simulink model "EOM_oceancurrents"  (R2023b)
settings: Solver=ode45  StartTime=0.0  StopTime=100  RelTol=1e-3
values from neighbouring files (symbols this model uses):
  beta_w = 0    [EOM_input.m]
  CM = 2.909*10^-5    (= 2.909e-05)    [dcdata.m]
  flow = [a_c;b_c;speed_c]    [EOM_input.m]
  Jm = 6.24*10^-4    (= 0.000624)    [dcdata.m]
  Kb = 1.7629*10^-2    (= 0.017629)    [dcdata.m]
  Kt = 1.7629*10^-2    (= 0.017629)    [dcdata.m]
  La = 0.28    [dcdata.m]
  M = M_a + M_rb    [EOM_input.m]    (also in Mechatronics (1).m; Mechatronics.m)
  Ra = 0.22680    (= 0.2268)    [dcdata.m]
  tau_r = -T1*cos(alpha1)*0.065+T2*cos(alpha1)*0.35+T2*cos(alpha2)-T2*sin(alpha2)+Tb*0.35    [EOM_input.m]    (also in Mechatronics (1).m; Mechatronics.m)
  tau_u = T1*cos(alpha1)+T2*cos(alpha2)    [EOM_input.m]    (also in Mechatronics (1).m; Mechatronics.m)
  tau_v = T1*sin(alpha1)+T2*sin(alpha2)+Tb    [EOM_input.m]    (also in Mechatronics (1).m = T1*sin(alpha1)+T2*sin(alpha2); Mechatronics.m)
  Trat = Ia*Kt    (= 0.158661)    [dcdata.m]
  vw = 0    [EOM_input.m]
  wm = 564.9    [dcdata.m]
undefined symbols (not defined in the file or in its folder): current_magnitude_percentage, eta_req_global, eta_start_local, T_all
libraries: slpidlib x5
settings Model: Creator=helle  LastModifiedBy=chris

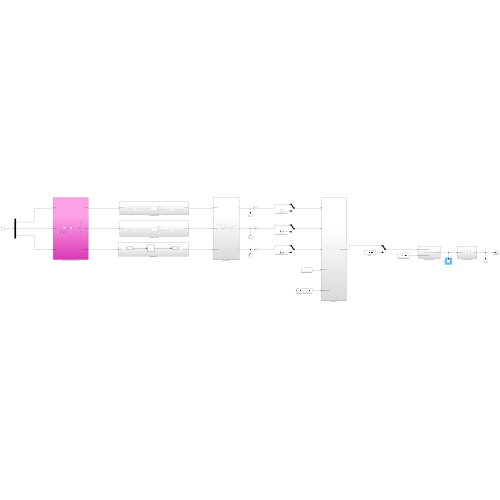
[thumbnail: Simulink's stored preview of the top-level diagram]
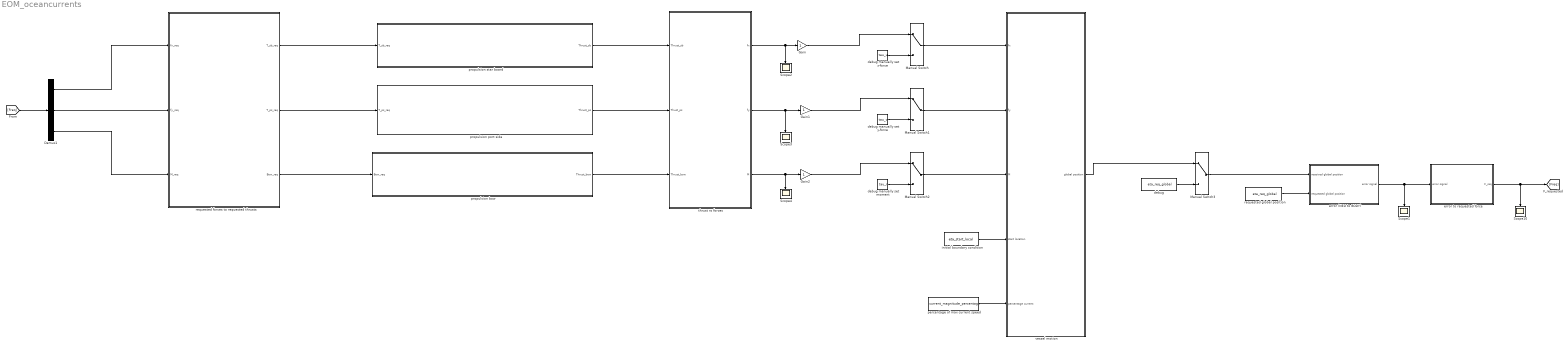
== system EOM_oceancurrents ==
  Demux1 : Demux  Outputs=3
  Gain : Gain
  Gain1 : Gain
  Gain2 : Gain
  Manual Switch{,1..3} (4 alike) : ManualSwitch
  Scope{1..4,10} (5 alike) : Scope
  debug : Constant  Value=eta_req_global
  debug manually set moment : Constant  Value=tau_r
  debug manually set x-force : Constant  Value=tau_u
  debug manually set y-force : Constant  Value=tau_v
  error (NED to BODY) : Subsystem
  error to requested force : Subsystem
  initial boundary condition : Constant  Value=eta_start_local
  percentage of max current speed : Constant  Value=current_magnitude_percentage
  propulsion bow : Subsystem
  propulsion port side : Subsystem
  propulsion star board : Subsystem
  requested forces to requested thrusts : Subsystem
  requested global position : Constant  Value=eta_req_global
  thrust ro forces : Subsystem
  vessel motion : Subsystem
  wires:
  Demux1/1 -> requested forces to requested thrusts/1(fx_req)
  Demux1/2 -> requested forces to requested thrusts/2(fy_req)
  Demux1/3 -> requested forces to requested thrusts/3(M_req)
  error to requested force/1(F_req) -> Scope10/1, [Freq]
  error (NED to BODY)/1(error signal) -> Scope1/1, error to requested force/1(error signal)
  thrust ro forces/1(fx) -> Scope2/1, Gain/1
  thrust ro forces/2(fy) -> Scope3/1, Gain1/1
  thrust ro forces/3(M) -> Scope4/1, Gain2/1
  propulsion bow/1(Thrust_bow) -> thrust ro forces/3(Thrust_bow)
  propulsion port side/1(Thrust_ps) -> thrust ro forces/2(Thust_ps)
  propulsion star board/1(Thrust_sb) -> thrust ro forces/1(Thrust_sb)
  requested forces to requested thrusts/1(T_sb_req) -> propulsion star board/1(T_sb_req)
  requested forces to requested thrusts/2(T_ps_req) -> propulsion port side/1(T_ps_req)
  requested forces to requested thrusts/3(Bow_req) -> propulsion bow/1(Bow_req)
  requested global position/1 -> error (NED to BODY)/2(requested global position)
  initial boundary condition/1 -> vessel motion/4(start location)
  [Freq] -> Demux1/1
  percentage of max current speed/1 -> vessel motion/5(percentage current)
  Manual Switch/1 -> vessel motion/1(fx)
  Gain/1 -> Manual Switch/1
  Manual Switch1/1 -> vessel motion/2(fy)
  Manual Switch2/1 -> vessel motion/3(M)
  Gain1/1 -> Manual Switch1/1
  Gain2/1 -> Manual Switch2/1
  debug manually set x-force/1 -> Manual Switch/2
  debug manually set y-force/1 -> Manual Switch1/2
  debug manually set moment/1 -> Manual Switch2/2
  Manual Switch3/1 -> error (NED to BODY)/1("received global position ")
  vessel motion/1(global position) -> Manual Switch3/1
  debug/1 -> Manual Switch3/2

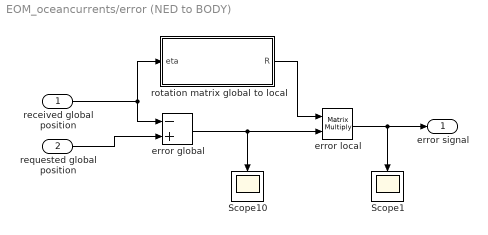
== system EOM_oceancurrents/error (NED to BODY) ==
  "received global position " : Inport
  requested global position : Inport  Port=2
  Scope1 : Scope
  Scope10 : Scope
  error global : Sum  Inputs=-+
  error local : Product  Multiplication=Matrix(*)
  rotation matrix global to local : MATLAB Function  TreatAsAtomicUnit=on
  error signal : Outport
  wires:
  "received global position "/1 -> rotation matrix global to local/1(eta), error global/1
  rotation matrix global to local/1(R) -> error local/1
  error local/1 -> Scope1/1, error signal/1
  requested global position/1 -> error global/2
  error global/1 -> Scope10/1, error local/2

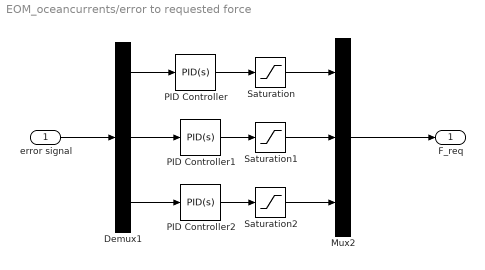
== system EOM_oceancurrents/error to requested force ==
  error signal : Inport
  Demux1 : Demux  Outputs=3
  Mux2 : Mux  Inputs=3
  PID Controller : slpidlib/PID Controller  Controller=PID  Form=Parallel  TimeDomain=Continuous-time  UseExternalTs=off  SampleTime=-1  IntegratorMethod=Forward Euler  FilterMethod=Forward Euler  ControllerParametersSource=internal  P=174.233635027511  I=4.06069558202177  UseKiTs=off  D=340.187698975111  N=319.667439985533  UseFilter=on  TunerSelectOption=Transfer Function Based (PID Tuner App)  InitialConditionSource=internal  InitialConditionForIntegrator=0  InitialConditionForFilter=0  DifferentiatorICPrevScaledInput=0  ExternalReset=none  TrackingMode=off  Kt=1  LimitOutput=off  SatLimitsSource=internal  UpperSaturationLimit=inf  LowerSaturationLimit=-inf  LinearizeAsGain=on  AntiWindupMode=none  Kb=1  LimitIntegrator=off  UpperIntegratorSaturationLimit=inf  LowerIntegratorSaturationLimit=-inf  POutMin=[]  POutMax=[]  IOutMin=[]  IOutMax=[]  DOutMin=[]  DOutMax=[]  NOutMin=[]  NOutMax=[]  SumOutMin=[]  SumOutMax=[]  SaturationOutMin=[]  SaturationOutMax=[]  PParamMin=[]  PParamMax=[]  IParamMin=[]  IParamMax=[]  DParamMin=[]  DParamMax=[]  NParamMin=[]  NParamMax=[]  KbParamMin=[]  KbParamMax=[]  KtParamMin=[]  KtParamMax=[]  KbOutMin=[]  KbOutMax=[]  KtOutMin=[]  KtOutMax=[]  IntegratorOutMin=[]  IntegratorOutMax=[]  FilterOutMin=[]  FilterOutMax=[]  SumI1OutMin=[]  SumI1OutMax=[]  SumI2OutMin=[]  SumI2OutMax=[]  SumI3OutMin=[]  SumI3OutMax=[]  SumI4OutMin=[]  SumI4OutMax=[]  SumDOutMin=[]  SumDOutMax=[]  DifferentiatorOutMin=[]  DifferentiatorOutMax=[]  FilterDiffOutCoefMin=[]  FilterDiffOutCoefMax=[]  ReciprocalOutMin=[]  ReciprocalOutMax=[]  SumDenOutMin=[]  SumDenOutMax=[]  SumNumOutMin=[]  SumNumOutMax=[]  DivideOutMin=[]  DivideOutMax=[]  UdiffTsProdOutMin=[]  UdiffTsProdOutMax=[]  NTsProdOutMin=[]  NTsProdOutMax=[]  UintegralTsProdOutMin=[]  UintegralTsProdOutMax=[]  UngainTsProdOutMin=[]  UngainTsProdOutMax=[]  ClampingZeroOutDataTypeStr=Inherit: Inherit via back propagation  ClampingZeroOutMin=[]  ClampingZeroOutMax=[]  FilterDenConstantOutDataTypeStr=Inherit: Inherit via back propagation  FilterDenConstantOutMin=[]  FilterDenConstantOutMax=[]  PCopyOutDataTypeStr=Inherit: Inherit via back propagation  PCopyOutMin=[]  PCopyOutMax=[]  NCopyOutDataTypeStr=Inherit: Inherit via back propagation  NCopyOutMin=[]  NCopyOutMax=[]  IntegratorContinuousStateAttributes=''  IntegratorStateMustResolveToSignalObject=off  IntegratorRTWStateStorageClass=Auto  FilterContinuousStateAttributes=''  FilterStateMustResolveToSignalObject=off  FilterRTWStateStorageClass=Auto  ParallelPVariant=InternalParameters  IdealPVariant=Disabled  IVariant=InternalParameters  DVariant=InternalParameters  IntegratorVariant=Continuous  SatVariant=Disabled  AWVariant=Passthrough  PCopyVariant=Disabled  TRVariant=Disabled  FdbkBlocksVariant=Forward  IdealPFdbkVariant=Disabled  SatFdbkVariant=Disabled  DerivativeFilterVariant=ContFilter  NVariant=InternalParameters  NCopyVariant=Disabled  FilterICVariant=InternalICsFilter  IntegratorICVariant=InternalICs  ExternalResetVariant=Disabled  TRSumVariant=Passthrough  SumFdbkVariant=Disabled  SumVariant=Sum_PID  TsampFilterVariant=InternalTs  TsampNgainVariant=Passthrough  TsampIntegralVariant=Disabled_SignalSpec  ExternalSaturationOutDataTypeStr=Inherit: Same as second input
  PID Controller1 : slpidlib/PID Controller  Controller=PID  Form=Parallel  TimeDomain=Continuous-time  UseExternalTs=off  SampleTime=-1  IntegratorMethod=Forward Euler  FilterMethod=Forward Euler  ControllerParametersSource=internal  P=97592.719586186  I=747986.305690658  UseKiTs=off  D=3078.78047810734  N=541.472412487083  UseFilter=on  TunerSelectOption=Transfer Function Based (PID Tuner App)  InitialConditionSource=internal  InitialConditionForIntegrator=0  InitialConditionForFilter=0  DifferentiatorICPrevScaledInput=0  ExternalReset=none  TrackingMode=off  Kt=1  LimitOutput=off  SatLimitsSource=internal  UpperSaturationLimit=inf  LowerSaturationLimit=-inf  LinearizeAsGain=on  AntiWindupMode=none  Kb=1  LimitIntegrator=off  UpperIntegratorSaturationLimit=inf  LowerIntegratorSaturationLimit=-inf  POutMin=[]  POutMax=[]  IOutMin=[]  IOutMax=[]  DOutMin=[]  DOutMax=[]  NOutMin=[]  NOutMax=[]  SumOutMin=[]  SumOutMax=[]  SaturationOutMin=[]  SaturationOutMax=[]  PParamMin=[]  PParamMax=[]  IParamMin=[]  IParamMax=[]  DParamMin=[]  DParamMax=[]  NParamMin=[]  NParamMax=[]  KbParamMin=[]  KbParamMax=[]  KtParamMin=[]  KtParamMax=[]  KbOutMin=[]  KbOutMax=[]  KtOutMin=[]  KtOutMax=[]  IntegratorOutMin=[]  IntegratorOutMax=[]  FilterOutMin=[]  FilterOutMax=[]  SumI1OutMin=[]  SumI1OutMax=[]  SumI2OutMin=[]  SumI2OutMax=[]  SumI3OutMin=[]  SumI3OutMax=[]  SumI4OutMin=[]  SumI4OutMax=[]  SumDOutMin=[]  SumDOutMax=[]  DifferentiatorOutMin=[]  DifferentiatorOutMax=[]  FilterDiffOutCoefMin=[]  FilterDiffOutCoefMax=[]  ReciprocalOutMin=[]  ReciprocalOutMax=[]  SumDenOutMin=[]  SumDenOutMax=[]  SumNumOutMin=[]  SumNumOutMax=[]  DivideOutMin=[]  DivideOutMax=[]  UdiffTsProdOutMin=[]  UdiffTsProdOutMax=[]  NTsProdOutMin=[]  NTsProdOutMax=[]  UintegralTsProdOutMin=[]  UintegralTsProdOutMax=[]  UngainTsProdOutMin=[]  UngainTsProdOutMax=[]  ClampingZeroOutDataTypeStr=Inherit: Inherit via back propagation  ClampingZeroOutMin=[]  ClampingZeroOutMax=[]  FilterDenConstantOutDataTypeStr=Inherit: Inherit via back propagation  FilterDenConstantOutMin=[]  FilterDenConstantOutMax=[]  PCopyOutDataTypeStr=Inherit: Inherit via back propagation  PCopyOutMin=[]  PCopyOutMax=[]  NCopyOutDataTypeStr=Inherit: Inherit via back propagation  NCopyOutMin=[]  NCopyOutMax=[]  IntegratorContinuousStateAttributes=''  IntegratorStateMustResolveToSignalObject=off  IntegratorRTWStateStorageClass=Auto  FilterContinuousStateAttributes=''  FilterStateMustResolveToSignalObject=off  FilterRTWStateStorageClass=Auto  ParallelPVariant=InternalParameters  IdealPVariant=Disabled  IVariant=InternalParameters  DVariant=InternalParameters  IntegratorVariant=Continuous  SatVariant=Disabled  AWVariant=Passthrough  PCopyVariant=Disabled  TRVariant=Disabled  FdbkBlocksVariant=Forward  IdealPFdbkVariant=Disabled  SatFdbkVariant=Disabled  DerivativeFilterVariant=ContFilter  NVariant=InternalParameters  NCopyVariant=Disabled  FilterICVariant=InternalICsFilter  IntegratorICVariant=InternalICs  ExternalResetVariant=Disabled  TRSumVariant=Passthrough  SumFdbkVariant=Disabled  SumVariant=Sum_PID  TsampFilterVariant=InternalTs  TsampNgainVariant=Passthrough  TsampIntegralVariant=Disabled_SignalSpec  ExternalSaturationOutDataTypeStr=Inherit: Same as second input
  PID Controller2 : slpidlib/PID Controller  Controller=PID  Form=Parallel  TimeDomain=Continuous-time  UseExternalTs=off  SampleTime=-1  IntegratorMethod=Forward Euler  FilterMethod=Forward Euler  ControllerParametersSource=internal  P=10.3561114578664  I=0.45191825910223  UseKiTs=off  D=53.5979577299415  N=151.545098117795  UseFilter=on  TunerSelectOption=Transfer Function Based (PID Tuner App)  InitialConditionSource=internal  InitialConditionForIntegrator=0  InitialConditionForFilter=0  DifferentiatorICPrevScaledInput=0  ExternalReset=none  TrackingMode=off  Kt=1  LimitOutput=off  SatLimitsSource=internal  UpperSaturationLimit=inf  LowerSaturationLimit=-inf  LinearizeAsGain=on  AntiWindupMode=none  Kb=1  LimitIntegrator=off  UpperIntegratorSaturationLimit=inf  LowerIntegratorSaturationLimit=-inf  POutMin=[]  POutMax=[]  IOutMin=[]  IOutMax=[]  DOutMin=[]  DOutMax=[]  NOutMin=[]  NOutMax=[]  SumOutMin=[]  SumOutMax=[]  SaturationOutMin=[]  SaturationOutMax=[]  PParamMin=[]  PParamMax=[]  IParamMin=[]  IParamMax=[]  DParamMin=[]  DParamMax=[]  NParamMin=[]  NParamMax=[]  KbParamMin=[]  KbParamMax=[]  KtParamMin=[]  KtParamMax=[]  KbOutMin=[]  KbOutMax=[]  KtOutMin=[]  KtOutMax=[]  IntegratorOutMin=[]  IntegratorOutMax=[]  FilterOutMin=[]  FilterOutMax=[]  SumI1OutMin=[]  SumI1OutMax=[]  SumI2OutMin=[]  SumI2OutMax=[]  SumI3OutMin=[]  SumI3OutMax=[]  SumI4OutMin=[]  SumI4OutMax=[]  SumDOutMin=[]  SumDOutMax=[]  DifferentiatorOutMin=[]  DifferentiatorOutMax=[]  FilterDiffOutCoefMin=[]  FilterDiffOutCoefMax=[]  ReciprocalOutMin=[]  ReciprocalOutMax=[]  SumDenOutMin=[]  SumDenOutMax=[]  SumNumOutMin=[]  SumNumOutMax=[]  DivideOutMin=[]  DivideOutMax=[]  UdiffTsProdOutMin=[]  UdiffTsProdOutMax=[]  NTsProdOutMin=[]  NTsProdOutMax=[]  UintegralTsProdOutMin=[]  UintegralTsProdOutMax=[]  UngainTsProdOutMin=[]  UngainTsProdOutMax=[]  ClampingZeroOutDataTypeStr=Inherit: Inherit via back propagation  ClampingZeroOutMin=[]  ClampingZeroOutMax=[]  FilterDenConstantOutDataTypeStr=Inherit: Inherit via back propagation  FilterDenConstantOutMin=[]  FilterDenConstantOutMax=[]  PCopyOutDataTypeStr=Inherit: Inherit via back propagation  PCopyOutMin=[]  PCopyOutMax=[]  NCopyOutDataTypeStr=Inherit: Inherit via back propagation  NCopyOutMin=[]  NCopyOutMax=[]  IntegratorContinuousStateAttributes=''  IntegratorStateMustResolveToSignalObject=off  IntegratorRTWStateStorageClass=Auto  FilterContinuousStateAttributes=''  FilterStateMustResolveToSignalObject=off  FilterRTWStateStorageClass=Auto  ParallelPVariant=InternalParameters  IdealPVariant=Disabled  IVariant=InternalParameters  DVariant=InternalParameters  IntegratorVariant=Continuous  SatVariant=Disabled  AWVariant=Passthrough  PCopyVariant=Disabled  TRVariant=Disabled  FdbkBlocksVariant=Forward  IdealPFdbkVariant=Disabled  SatFdbkVariant=Disabled  DerivativeFilterVariant=ContFilter  NVariant=InternalParameters  NCopyVariant=Disabled  FilterICVariant=InternalICsFilter  IntegratorICVariant=InternalICs  ExternalResetVariant=Disabled  TRSumVariant=Passthrough  SumFdbkVariant=Disabled  SumVariant=Sum_PID  TsampFilterVariant=InternalTs  TsampNgainVariant=Passthrough  TsampIntegralVariant=Disabled_SignalSpec  ExternalSaturationOutDataTypeStr=Inherit: Same as second input
  Saturation : Saturate  UpperLimit=2.5  LowerLimit=-2.5
  Saturation1 : Saturate  UpperLimit=2.5  LowerLimit=-2.5
  Saturation2 : Saturate  UpperLimit=2.5  LowerLimit=-2.5
  F_req : Outport
  wires:
  error signal/1 -> Demux1/1
  Demux1/1 -> PID Controller/1
  PID Controller1/1 -> Saturation1/1
  Saturation/1 -> Mux2/1
  Saturation2/1 -> Mux2/3
  Mux2/1 -> F_req/1
  PID Controller/1 -> Saturation/1
  Demux1/2 -> PID Controller1/1
  Saturation1/1 -> Mux2/2
  Demux1/3 -> PID Controller2/1
  PID Controller2/1 -> Saturation2/1

== system EOM_oceancurrents/propulsion bow ==
  Bow_req : Inport
  Saturation : Saturate  UpperLimit=2  LowerLimit=-2
  Thrust_bow : Outport
  wires:
  Saturation/1 -> Thrust_bow/1
  Bow_req/1 -> Saturation/1

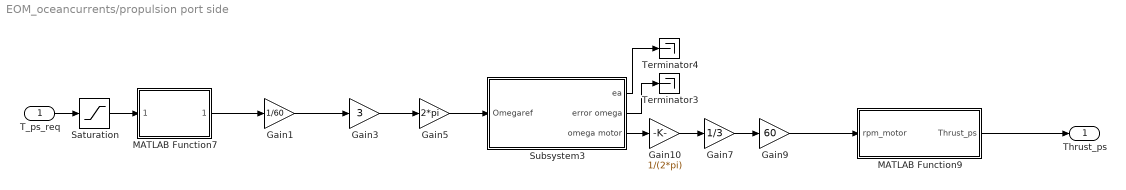
== system EOM_oceancurrents/propulsion port side ==
  T_ps_req : Inport
  Gain1 : Gain  Gain=1/60
  Gain10 : Gain  Gain=1/(2*pi)
  Gain3 : Gain  Gain=3
  Gain5 : Gain  Gain=2*pi
  Gain7 : Gain  Gain=1/3
  Gain9 : Gain  Gain=60
  MATLAB Function7 : MATLAB Function  TreatAsAtomicUnit=on
  MATLAB Function9 : MATLAB Function  TreatAsAtomicUnit=on
  Saturation : Saturate  UpperLimit=3  LowerLimit=-3
  Subsystem3 : Subsystem
  Terminator3 : Terminator
  Terminator4 : Terminator
  Thrust_ps : Outport
  wires:
  Gain9/1 -> MATLAB Function9/1(rpm_motor)
  T_ps_req/1 -> Saturation/1
  Gain5/1 -> Subsystem3/1(Omegaref)
  Gain10/1 -> Gain7/1
  Gain7/1 -> Gain9/1
  Gain3/1 -> Gain5/1
  MATLAB Function7/1(rpmreq) -> Gain1/1
  Subsystem3/3(omega motor) -> Gain10/1
  MATLAB Function9/1(Thrust_ps) -> Thrust_ps/1
  Gain1/1 -> Gain3/1
  Subsystem3/2(error omega) -> Terminator3/1
  Subsystem3/1(ea) -> Terminator4/1
  Saturation/1 -> MATLAB Function7/1(T_ps_req)

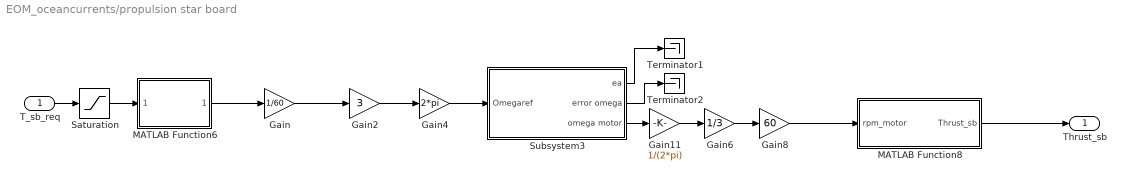
== system EOM_oceancurrents/propulsion star board ==
  T_sb_req : Inport
  Gain : Gain  Gain=1/60
  Gain11 : Gain  Gain=1/(2*pi)
  Gain2 : Gain  Gain=3
  Gain4 : Gain  Gain=2*pi
  Gain6 : Gain  Gain=1/3
  Gain8 : Gain  Gain=60
  MATLAB Function6 : MATLAB Function  TreatAsAtomicUnit=on
  MATLAB Function8 : MATLAB Function  TreatAsAtomicUnit=on
  Saturation : Saturate  UpperLimit=3  LowerLimit=-3
  Subsystem3 : Subsystem
  Terminator1 : Terminator
  Terminator2 : Terminator
  Thrust_sb : Outport
  wires:
  MATLAB Function6/1(rpmreq) -> Gain/1
  T_sb_req/1 -> Saturation/1
  Subsystem3/3(omega motor) -> Gain11/1
  Gain6/1 -> Gain8/1
  Subsystem3/1(ea) -> Terminator1/1
  Gain2/1 -> Gain4/1
  Gain11/1 -> Gain6/1
  Gain4/1 -> Subsystem3/1(Omegaref)
  Gain/1 -> Gain2/1
  MATLAB Function8/1(Thrust_sb) -> Thrust_sb/1
  Gain8/1 -> MATLAB Function8/1(rpm_motor)
  Subsystem3/2(error omega) -> Terminator2/1
  Saturation/1 -> MATLAB Function6/1(T_sb_req)

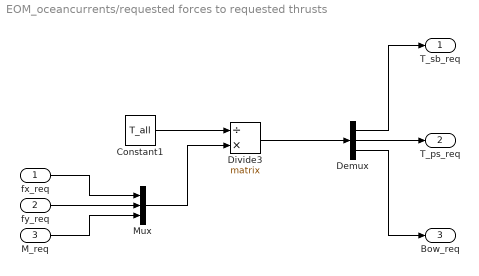
== system EOM_oceancurrents/requested forces to requested thrusts ==
  fx_req : Inport
  fy_req : Inport  Port=2
  M_req : Inport  Port=3
  Constant1 : Constant  Value=T_all
  Demux : Demux  Outputs=3
  Divide3 : Product  Inputs=/*  Multiplication=Matrix(*)
  Mux : Mux  Inputs=3
  T_sb_req : Outport
  T_ps_req : Outport  Port=2
  Bow_req : Outport  Port=3
  wires:
  Demux/1 -> T_sb_req/1
  Mux/1 -> Divide3/2
  Demux/3 -> Bow_req/1
  M_req/1 -> Mux/3
  fy_req/1 -> Mux/2
  Divide3/1 -> Demux/1
  Demux/2 -> T_ps_req/1
  Constant1/1 -> Divide3/1
  fx_req/1 -> Mux/1

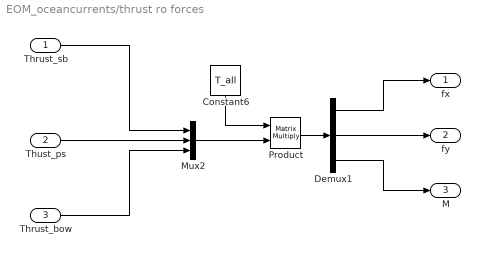
== system EOM_oceancurrents/thrust ro forces ==
  Thrust_sb : Inport
  Thust_ps : Inport  Port=2
  Thrust_bow : Inport  Port=3
  Constant6 : Constant  Value=T_all
  Demux1 : Demux  Outputs=3
  Mux2 : Mux  Inputs=3
  Product : Product  Multiplication=Matrix(*)
  fx : Outport
  fy : Outport  Port=2
  M : Outport  Port=3
  wires:
  Thrust_bow/1 -> Mux2/3
  Thrust_sb/1 -> Mux2/1
  Demux1/1 -> fx/1
  Mux2/1 -> Product/2
  Thust_ps/1 -> Mux2/2
  Demux1/3 -> M/1
  Demux1/2 -> fy/1
  Constant6/1 -> Product/1
  Product/1 -> Demux1/1

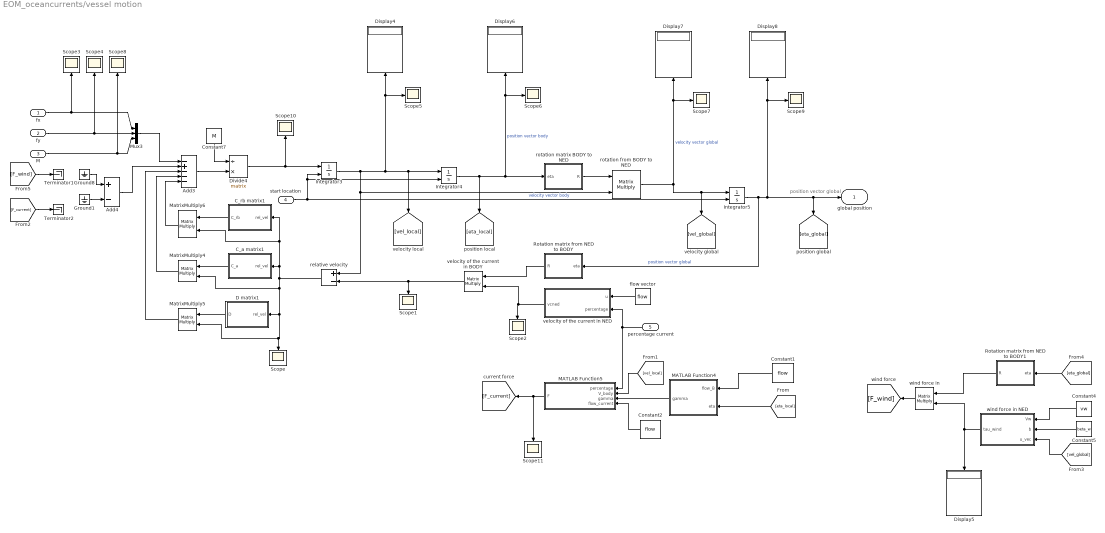
== system EOM_oceancurrents/vessel motion ==
  note: position vector global
  fx : Inport
  fy : Inport  Port=2
  M : Inport  Port=3
  start location : Inport  Port=4
  percentage current : Inport  Port=5
  Add3 : Sum  Inputs=-+---
  Add4 : Sum  Inputs=+-
  C_a matrix1 : MATLAB Function  TreatAsAtomicUnit=on
  C_rb matrix1 : MATLAB Function  TreatAsAtomicUnit=on
  Constant1 : Constant  Value=flow
  Constant2 : Constant  Value=flow
  Constant4 : Constant  Value=vw
  Constant5 : Constant  Value=beta_w
  Constant7 : Constant  Value=M
  D matrix1 : MATLAB Function  TreatAsAtomicUnit=on
  Display{4..8} (5 alike) : Display
  Divide4 : Product  Inputs=/*  Multiplication=Matrix(*)
  Ground1 : Ground
  Ground8 : Ground
  Integrator3 : Integrator  InitialConditionSource=external
  Integrator4 : Integrator  InitialConditionSource=external
  Integrator5 : Integrator  InitialConditionSource=external
  MATLAB Function4 : MATLAB Function  TreatAsAtomicUnit=on
  MATLAB Function5 : MATLAB Function  TreatAsAtomicUnit=on
  MatrixMultiply4 : Product  Multiplication=Matrix(*)
  MatrixMultiply5 : Product  Multiplication=Matrix(*)
  MatrixMultiply6 : Product  Multiplication=Matrix(*)
  Mux3 : Mux  Inputs=3
  Rotation matrix from NED to BODY : MATLAB Function  TreatAsAtomicUnit=on
  Rotation matrix from NED to BODY1 : MATLAB Function  TreatAsAtomicUnit=on
  Scope{,1..11} (12 alike) : Scope
  Terminator1 : Terminator
  Terminator2 : Terminator
  flow vector : Constant  Value=flow
  relative velocity : Sum  Inputs=+-
  rotation from BODY to NED : Product  Multiplication=Matrix(*)
  rotation matrix BODY to NED : MATLAB Function  TreatAsAtomicUnit=on
  velocity of the current in BODY : Product  Inputs=**  Multiplication=Matrix(*)
  velocity of the current in NED : MATLAB Function  TreatAsAtomicUnit=on
  "wind force in " : Product  Inputs=**  Multiplication=Matrix(*)
  wind force in NED : MATLAB Function  TreatAsAtomicUnit=on
  global position : Outport
  wires:
  Integrator3/1 -> Scope5/1, Display4/1, [vel_local], Integrator4/1, relative velocity/1, rotation from BODY to NED/2  "velocity vector body"
  rotation from BODY to NED/1 -> Scope7/1, Display7/1, [vel_global], Integrator5/1  "velocity vector global"
  Divide4/1 -> Scope10/1, Integrator3/1
  relative velocity/1 -> Scope/1, MatrixMultiply5/2, D matrix1/1(rel_vel), MatrixMultiply4/2, C_a matrix1/1(rel_vel), C_rb matrix1/1(rel_vel), MatrixMultiply6/2
  Integrator5/1 -> [eta_global], global position/1, Display8/1, Scope9/1, Rotation matrix from NED to BODY/1(eta)  "position vector global"
  Integrator4/1 -> Scope6/1, Display6/1, rotation matrix BODY to NED/1(eta), [eta_local]  "position vector body"
  C_rb matrix1/1(C_rb) -> MatrixMultiply6/1
  Ground8/1 -> Add4/1
  MatrixMultiply4/1 -> Add3/4
  MatrixMultiply6/1 -> Add3/5
  rotation matrix BODY to NED/1(R) -> rotation from BODY to NED/1
  D matrix1/1(D) -> MatrixMultiply5/1
  C_a matrix1/1(C_a) -> MatrixMultiply4/1
  Mux3/1 -> Add3/1
  MatrixMultiply5/1 -> Add3/3
  Rotation matrix from NED to BODY/1(R) -> velocity of the current in BODY/1
  Constant7/1 -> Divide4/1
  Add3/1 -> Divide4/2
  Add4/1 -> Add3/2
  flow vector/1 -> velocity of the current in NED/1(u)
  velocity of the current in BODY/1 -> Scope1/1, relative velocity/2
  fy/1 -> Scope4/1, Mux3/2
  fx/1 -> Scope3/1, Mux3/1
  M/1 -> Scope8/1, Mux3/3
  MATLAB Function4/1(gamma) -> MATLAB Function5/3(gamma)
  [eta_local] -> MATLAB Function4/2(eta)
  Constant1/1 -> MATLAB Function4/1(flow_B)
  Constant2/1 -> MATLAB Function5/4(flow_current)
  [vel_local] -> MATLAB Function5/2(V_body)
  MATLAB Function5/1(F) -> Scope11/1, [F_current]
  velocity of the current in NED/1(vcned) -> Scope2/1, velocity of the current in BODY/2
  Constant4/1 -> wind force in NED/1(Vw)
  "wind force in "/1 -> [F_wind]
  Constant5/1 -> wind force in NED/2(b)
  wind force in NED/1(tau_wind) -> Display5/1, "wind force in "/2
  [vel_global] -> wind force in NED/3(u_vec)
  [eta_global] -> Rotation matrix from NED to BODY1/1(eta)
  Rotation matrix from NED to BODY1/1(R) -> "wind force in "/1
  [F_wind] -> Terminator1/1
  start location/1 -> Integrator3/2, Integrator4/2, Integrator5/2
  percentage current/1 -> velocity of the current in NED/2(percentage), MATLAB Function5/1(percentage)
  [F_current] -> Terminator2/1
  Ground1/1 -> Add4/2

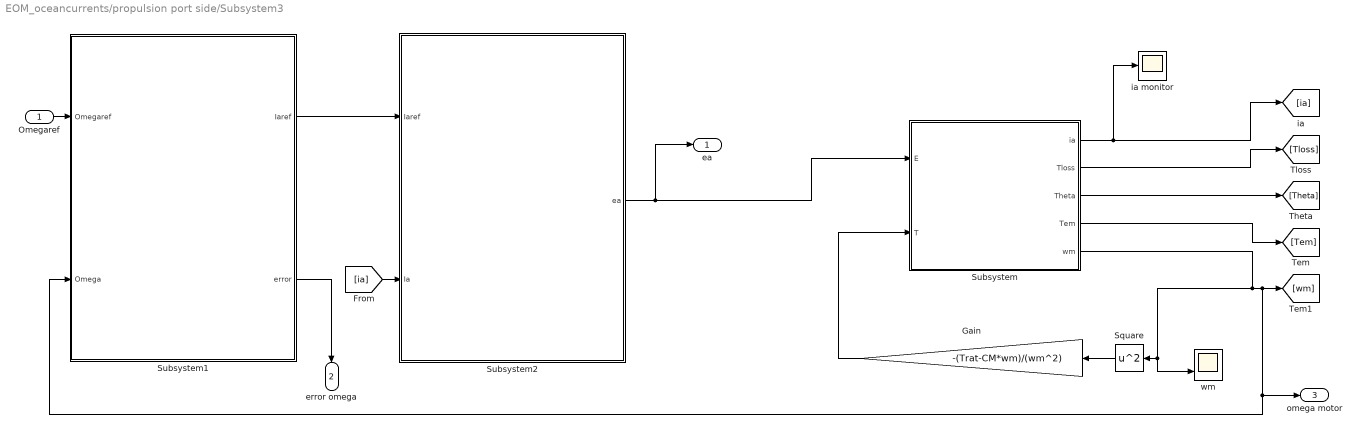
== system EOM_oceancurrents/propulsion port side/Subsystem3 ==
  Omegaref : Inport
  Gain : Gain  Gain=-(Trat-CM*wm)/(wm^2)
  Square : Math  Operator=square
  Subsystem : Subsystem
  Subsystem1 : Subsystem
  Subsystem2 : Subsystem
  ia monitor : Scope
  wm : Scope  NumInputPorts=2
  ea : Outport
  error omega : Outport  Port=2
  omega motor : Outport  Port=3
  wires:
  Subsystem/5(wm) -> omega motor/1, Subsystem1/2(Omega), [wm], Square/1, wm/2
  Gain/1 -> Subsystem/2(T)
  Subsystem/1(ia) -> ia monitor/1, [ia]
  Subsystem1/1(Iaref) -> Subsystem2/1(Iaref)
  Subsystem1/2(error) -> error omega/1
  Square/1 -> Gain/1
  Omegaref/1 -> Subsystem1/1(Omegaref)
  Subsystem2/1(ea) -> Subsystem/1(E), ea/1
  Subsystem/2(Tloss) -> [Tloss]
  Subsystem/3(Theta) -> [Theta]
  Subsystem/4(Tem) -> [Tem]
  [ia] -> Subsystem2/2(Ia)

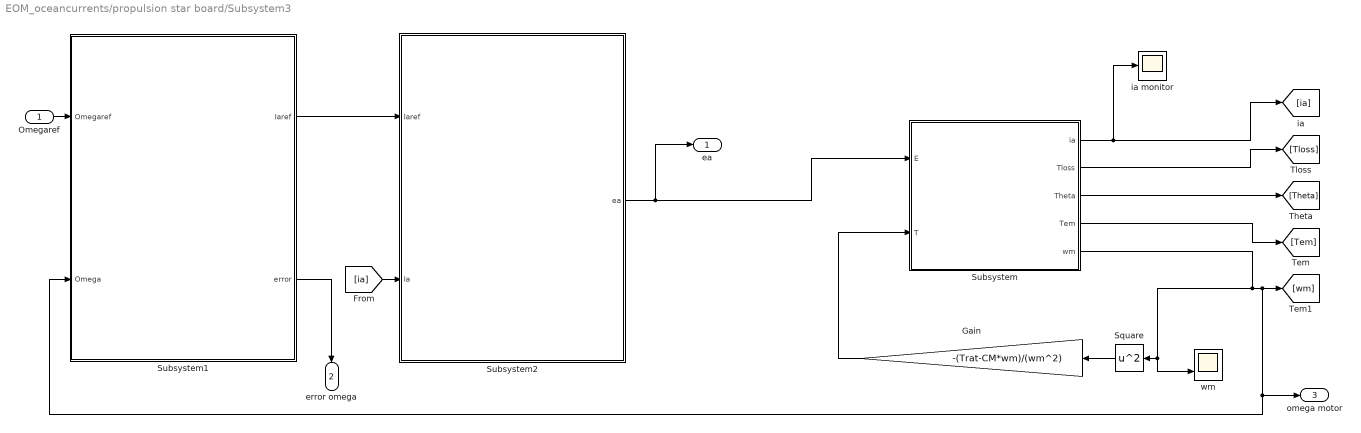
== system EOM_oceancurrents/propulsion star board/Subsystem3 ==
  Omegaref : Inport
  Gain : Gain  Gain=-(Trat-CM*wm)/(wm^2)
  Square : Math  Operator=square
  Subsystem : Subsystem
  Subsystem1 : Subsystem
  Subsystem2 : Subsystem
  ia monitor : Scope
  wm : Scope  NumInputPorts=2
  ea : Outport
  error omega : Outport  Port=2
  omega motor : Outport  Port=3
  wires:
  Subsystem/5(wm) -> omega motor/1, Subsystem1/2(Omega), [wm], Square/1, wm/2
  Gain/1 -> Subsystem/2(T)
  Subsystem/1(ia) -> ia monitor/1, [ia]
  Subsystem1/1(Iaref) -> Subsystem2/1(Iaref)
  Subsystem1/2(error) -> error omega/1
  Square/1 -> Gain/1
  Omegaref/1 -> Subsystem1/1(Omegaref)
  Subsystem2/1(ea) -> Subsystem/1(E), ea/1
  Subsystem/2(Tloss) -> [Tloss]
  Subsystem/3(Theta) -> [Theta]
  Subsystem/4(Tem) -> [Tem]
  [ia] -> Subsystem2/2(Ia)

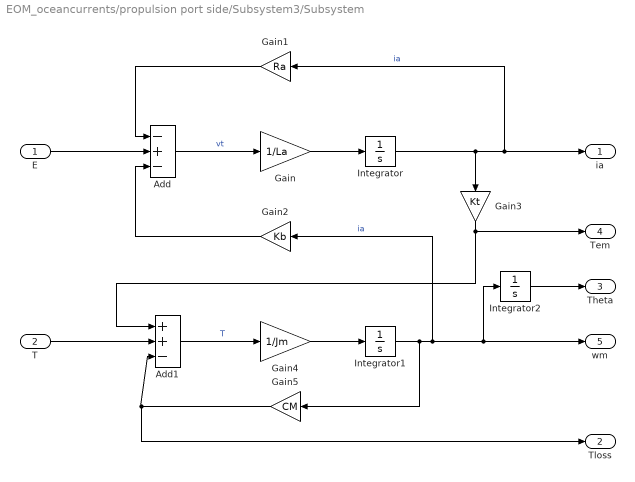
== system EOM_oceancurrents/propulsion port side/Subsystem3/Subsystem ==
  E : Inport
  T : Inport  Port=2
  Add : Sum  Inputs=-+-
  Add1 : Sum  Inputs=++-
  Gain : Gain  Gain=1/La
  Gain1 : Gain  Gain=Ra
  Gain2 : Gain  Gain=Kb
  Gain3 : Gain  Gain=Kt
  Gain4 : Gain  Gain=1/Jm
  Gain5 : Gain  Gain=CM
  Integrator : Integrator
  Integrator1 : Integrator
  Integrator2 : Integrator
  ia : Outport
  Tloss : Outport  Port=2
  Theta : Outport  Port=3
  Tem : Outport  Port=4
  wm : Outport  Port=5
  wires:
  Gain2/1 -> Add/3
  Gain/1 -> Integrator/1
  Integrator1/1 -> wm/1, Integrator2/1, Gain2/1, Gain5/1  "ia"
  Add1/1 -> Gain4/1  "T"
  Add/1 -> Gain/1  "vt"
  Gain1/1 -> Add/1
  Gain4/1 -> Integrator1/1
  Integrator/1 -> ia/1, Gain1/1, Gain3/1  "ia"
  Gain3/1 -> Add1/1, Tem/1
  Gain5/1 -> Tloss/1, Add1/3
  E/1 -> Add/2
  T/1 -> Add1/2
  Integrator2/1 -> Theta/1

== system EOM_oceancurrents/propulsion port side/Subsystem3/Subsystem1 ==
  Omegaref : Inport
  Omega : Inport  Port=2
  Add : Sum  Inputs=+-
  Gain : Gain  Gain=1/wm
  PID Controller : slpidlib/PID Controller  Controller=PID  Form=Ideal  TimeDomain=Continuous-time  UseExternalTs=off  SampleTime=-1  IntegratorMethod=Forward Euler  FilterMethod=Forward Euler  ControllerParametersSource=internal  P=99.1419908148733  I=0.405774649898487  UseKiTs=off  D=0.0328385363334431  N=5.23608118750105  UseFilter=on  TunerSelectOption=Transfer Function Based (PID Tuner App)  InitialConditionSource=internal  InitialConditionForIntegrator=0  InitialConditionForFilter=0  DifferentiatorICPrevScaledInput=0  ExternalReset=none  TrackingMode=off  Kt=1  LimitOutput=off  SatLimitsSource=internal  UpperSaturationLimit=inf  LowerSaturationLimit=-inf  LinearizeAsGain=on  AntiWindupMode=none  Kb=1  LimitIntegrator=off  UpperIntegratorSaturationLimit=inf  LowerIntegratorSaturationLimit=-inf  POutMin=[]  POutMax=[]  IOutMin=[]  IOutMax=[]  DOutMin=[]  DOutMax=[]  NOutMin=[]  NOutMax=[]  SumOutMin=[]  SumOutMax=[]  SaturationOutMin=[]  SaturationOutMax=[]  PParamMin=[]  PParamMax=[]  IParamMin=[]  IParamMax=[]  DParamMin=[]  DParamMax=[]  NParamMin=[]  NParamMax=[]  KbParamMin=[]  KbParamMax=[]  KtParamMin=[]  KtParamMax=[]  KbOutMin=[]  KbOutMax=[]  KtOutMin=[]  KtOutMax=[]  IntegratorOutMin=[]  IntegratorOutMax=[]  FilterOutMin=[]  FilterOutMax=[]  SumI1OutMin=[]  SumI1OutMax=[]  SumI2OutMin=[]  SumI2OutMax=[]  SumI3OutMin=[]  SumI3OutMax=[]  SumI4OutMin=[]  SumI4OutMax=[]  SumDOutMin=[]  SumDOutMax=[]  DifferentiatorOutMin=[]  DifferentiatorOutMax=[]  FilterDiffOutCoefMin=[]  FilterDiffOutCoefMax=[]  ReciprocalOutMin=[]  ReciprocalOutMax=[]  SumDenOutMin=[]  SumDenOutMax=[]  SumNumOutMin=[]  SumNumOutMax=[]  DivideOutMin=[]  DivideOutMax=[]  UdiffTsProdOutMin=[]  UdiffTsProdOutMax=[]  NTsProdOutMin=[]  NTsProdOutMax=[]  UintegralTsProdOutMin=[]  UintegralTsProdOutMax=[]  UngainTsProdOutMin=[]  UngainTsProdOutMax=[]  ClampingZeroOutDataTypeStr=Inherit: Inherit via back propagation  ClampingZeroOutMin=[]  ClampingZeroOutMax=[]  FilterDenConstantOutDataTypeStr=Inherit: Inherit via back propagation  FilterDenConstantOutMin=[]  FilterDenConstantOutMax=[]  PCopyOutDataTypeStr=Inherit: Inherit via back propagation  PCopyOutMin=[]  PCopyOutMax=[]  NCopyOutDataTypeStr=Inherit: Inherit via back propagation  NCopyOutMin=[]  NCopyOutMax=[]  IntegratorContinuousStateAttributes=''  IntegratorStateMustResolveToSignalObject=off  IntegratorRTWStateStorageClass=Auto  FilterContinuousStateAttributes=''  FilterStateMustResolveToSignalObject=off  FilterRTWStateStorageClass=Auto  ParallelPVariant=Passthrough  IdealPVariant=InternalParameters  IVariant=InternalParameters  DVariant=InternalParameters  IntegratorVariant=Continuous  SatVariant=Disabled  AWVariant=Passthrough  PCopyVariant=Disabled  TRVariant=Disabled  FdbkBlocksVariant=Forward  IdealPFdbkVariant=Disabled  SatFdbkVariant=Disabled  DerivativeFilterVariant=ContFilter  NVariant=InternalParameters  NCopyVariant=Disabled  FilterICVariant=InternalICsFilter  IntegratorICVariant=InternalICs  ExternalResetVariant=Disabled  TRSumVariant=Passthrough  SumFdbkVariant=Disabled  SumVariant=Sum_PID  TsampFilterVariant=InternalTs  TsampNgainVariant=Passthrough  TsampIntegralVariant=Disabled_SignalSpec  ExternalSaturationOutDataTypeStr=Inherit: Same as second input
  Saturation : Saturate
  Iaref : Outport
  error : Outport  Port=2
  wires:
  Omegaref/1 -> Add/1
  Omega/1 -> Add/2
  Add/1 -> Gain/1
  Gain/1 -> PID Controller/1, error/1
  Saturation/1 -> Iaref/1
  PID Controller/1 -> Saturation/1

== system EOM_oceancurrents/propulsion port side/Subsystem3/Subsystem2 ==
  Iaref : Inport
  Ia : Inport  Port=2
  Add : Sum  Inputs=+-
  Transfer Fcn : TransferFcn  Numerator=[10]  Denominator=[0.1 1]
  ea : Outport
  wires:
  Iaref/1 -> Add/1
  Ia/1 -> Add/2
  Add/1 -> Transfer Fcn/1
  Transfer Fcn/1 -> ea/1

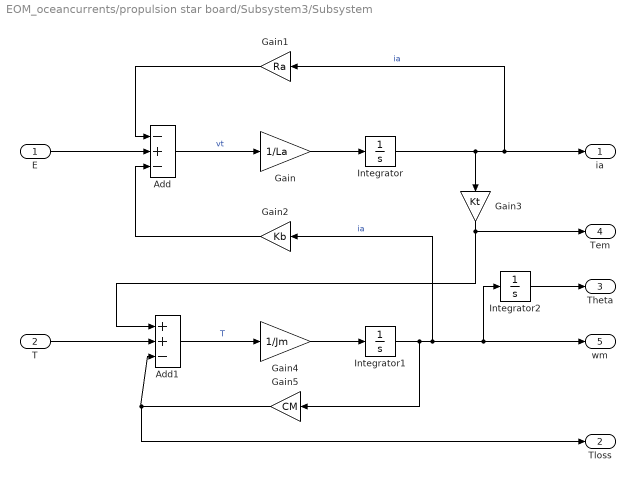
== system EOM_oceancurrents/propulsion star board/Subsystem3/Subsystem ==
  E : Inport
  T : Inport  Port=2
  Add : Sum  Inputs=-+-
  Add1 : Sum  Inputs=++-
  Gain : Gain  Gain=1/La
  Gain1 : Gain  Gain=Ra
  Gain2 : Gain  Gain=Kb
  Gain3 : Gain  Gain=Kt
  Gain4 : Gain  Gain=1/Jm
  Gain5 : Gain  Gain=CM
  Integrator : Integrator
  Integrator1 : Integrator
  Integrator2 : Integrator
  ia : Outport
  Tloss : Outport  Port=2
  Theta : Outport  Port=3
  Tem : Outport  Port=4
  wm : Outport  Port=5
  wires:
  Gain2/1 -> Add/3
  Gain/1 -> Integrator/1
  Integrator1/1 -> wm/1, Integrator2/1, Gain2/1, Gain5/1  "ia"
  Add1/1 -> Gain4/1  "T"
  Add/1 -> Gain/1  "vt"
  Gain1/1 -> Add/1
  Gain4/1 -> Integrator1/1
  Integrator/1 -> ia/1, Gain1/1, Gain3/1  "ia"
  Gain3/1 -> Add1/1, Tem/1
  Gain5/1 -> Tloss/1, Add1/3
  E/1 -> Add/2
  T/1 -> Add1/2
  Integrator2/1 -> Theta/1

== system EOM_oceancurrents/propulsion star board/Subsystem3/Subsystem1 ==
  Omegaref : Inport
  Omega : Inport  Port=2
  Add : Sum  Inputs=+-
  Gain : Gain  Gain=1/wm
  PID Controller : slpidlib/PID Controller  Controller=PID  Form=Ideal  TimeDomain=Continuous-time  UseExternalTs=off  SampleTime=-1  IntegratorMethod=Forward Euler  FilterMethod=Forward Euler  ControllerParametersSource=internal  P=99.1419908148733  I=0.405774649898487  UseKiTs=off  D=0.0328385363334431  N=5.23608118750105  UseFilter=on  TunerSelectOption=Transfer Function Based (PID Tuner App)  InitialConditionSource=internal  InitialConditionForIntegrator=0  InitialConditionForFilter=0  DifferentiatorICPrevScaledInput=0  ExternalReset=none  TrackingMode=off  Kt=1  LimitOutput=off  SatLimitsSource=internal  UpperSaturationLimit=inf  LowerSaturationLimit=-inf  LinearizeAsGain=on  AntiWindupMode=none  Kb=1  LimitIntegrator=off  UpperIntegratorSaturationLimit=inf  LowerIntegratorSaturationLimit=-inf  POutMin=[]  POutMax=[]  IOutMin=[]  IOutMax=[]  DOutMin=[]  DOutMax=[]  NOutMin=[]  NOutMax=[]  SumOutMin=[]  SumOutMax=[]  SaturationOutMin=[]  SaturationOutMax=[]  PParamMin=[]  PParamMax=[]  IParamMin=[]  IParamMax=[]  DParamMin=[]  DParamMax=[]  NParamMin=[]  NParamMax=[]  KbParamMin=[]  KbParamMax=[]  KtParamMin=[]  KtParamMax=[]  KbOutMin=[]  KbOutMax=[]  KtOutMin=[]  KtOutMax=[]  IntegratorOutMin=[]  IntegratorOutMax=[]  FilterOutMin=[]  FilterOutMax=[]  SumI1OutMin=[]  SumI1OutMax=[]  SumI2OutMin=[]  SumI2OutMax=[]  SumI3OutMin=[]  SumI3OutMax=[]  SumI4OutMin=[]  SumI4OutMax=[]  SumDOutMin=[]  SumDOutMax=[]  DifferentiatorOutMin=[]  DifferentiatorOutMax=[]  FilterDiffOutCoefMin=[]  FilterDiffOutCoefMax=[]  ReciprocalOutMin=[]  ReciprocalOutMax=[]  SumDenOutMin=[]  SumDenOutMax=[]  SumNumOutMin=[]  SumNumOutMax=[]  DivideOutMin=[]  DivideOutMax=[]  UdiffTsProdOutMin=[]  UdiffTsProdOutMax=[]  NTsProdOutMin=[]  NTsProdOutMax=[]  UintegralTsProdOutMin=[]  UintegralTsProdOutMax=[]  UngainTsProdOutMin=[]  UngainTsProdOutMax=[]  ClampingZeroOutDataTypeStr=Inherit: Inherit via back propagation  ClampingZeroOutMin=[]  ClampingZeroOutMax=[]  FilterDenConstantOutDataTypeStr=Inherit: Inherit via back propagation  FilterDenConstantOutMin=[]  FilterDenConstantOutMax=[]  PCopyOutDataTypeStr=Inherit: Inherit via back propagation  PCopyOutMin=[]  PCopyOutMax=[]  NCopyOutDataTypeStr=Inherit: Inherit via back propagation  NCopyOutMin=[]  NCopyOutMax=[]  IntegratorContinuousStateAttributes=''  IntegratorStateMustResolveToSignalObject=off  IntegratorRTWStateStorageClass=Auto  FilterContinuousStateAttributes=''  FilterStateMustResolveToSignalObject=off  FilterRTWStateStorageClass=Auto  ParallelPVariant=Passthrough  IdealPVariant=InternalParameters  IVariant=InternalParameters  DVariant=InternalParameters  IntegratorVariant=Continuous  SatVariant=Disabled  AWVariant=Passthrough  PCopyVariant=Disabled  TRVariant=Disabled  FdbkBlocksVariant=Forward  IdealPFdbkVariant=Disabled  SatFdbkVariant=Disabled  DerivativeFilterVariant=ContFilter  NVariant=InternalParameters  NCopyVariant=Disabled  FilterICVariant=InternalICsFilter  IntegratorICVariant=InternalICs  ExternalResetVariant=Disabled  TRSumVariant=Passthrough  SumFdbkVariant=Disabled  SumVariant=Sum_PID  TsampFilterVariant=InternalTs  TsampNgainVariant=Passthrough  TsampIntegralVariant=Disabled_SignalSpec  ExternalSaturationOutDataTypeStr=Inherit: Same as second input
  Saturation : Saturate
  Iaref : Outport
  error : Outport  Port=2
  wires:
  Omegaref/1 -> Add/1
  Omega/1 -> Add/2
  Add/1 -> Gain/1
  Gain/1 -> PID Controller/1, error/1
  Saturation/1 -> Iaref/1
  PID Controller/1 -> Saturation/1

== system EOM_oceancurrents/propulsion star board/Subsystem3/Subsystem2 ==
  Iaref : Inport
  Ia : Inport  Port=2
  Add : Sum  Inputs=+-
  Transfer Fcn : TransferFcn  Numerator=[10]  Denominator=[0.1 1]
  ea : Outport
  wires:
  Iaref/1 -> Add/1
  Ia/1 -> Add/2
  Add/1 -> Transfer Fcn/1
  Transfer Fcn/1 -> ea/1

== matlab function EOM_oceancurrents/propulsion star board/MATLAB Function6 ==
  data: rpmreq output; T_sb_req input
function rpmreq = fcn(T_sb_req)

rpmreq = -69.944*T_sb_req^3 + 15.905*T_sb_req^2 + 831.34*T_sb_req - 43.291;

== matlab function EOM_oceancurrents/vessel motion/wind force in NED ==
  data: Vw input; tau_wind output; b input; u_vec input
function tau_wind = fcn(Vw,b,u_vec)
rho_a =1.293;
B = 0.32;
Loa=0.97;
A_fw=0.8*B^2;
A_lw=Loa*B*0.8;
u=u_vec(1);
v=u_vec(2);
psi=u_vec(3);
uw=Vw*cos(b-psi);
vw=Vw*sin(b-psi);
urw=u-uw;
vrw=v-vw;
Vrw=(urw^2+vrw^2)^(1/2);
gammarw=-atan2(vrw,urw)*180/pi;
CX=(-8*10^(-7))*gammarw^3 + 0.0002*gammarw^2-0.0081*gammarw - 0.5206;
CY=(3*10^-12)*gammarw^6 - 2*10^-09*gammarw^5 + 4*10^-07*gammarw^4 - 4*10^-05*gammarw^3 + 0.0014*gammarw^2 - 0.0013*gammarw + 0.0291;
CN=-5*10^-11*gammarw^4 + 2*10^-07*gammarw^3 - 6*10^-05*gammarw^2 + 0.0042*gammarw + 0.0318;
%tau_wind = 0.5*rho_a*Vrw^2*[CX*A_fw;CY*A_lw;CN*A_lw*Loa];
tau_wind = [0;0;0];

== matlab function EOM_oceancurrents/vessel motion/Rotation matrix from NED to BODY1 ==
  data: eta input; R output
function R = fcn(eta)
psi=eta(3);

R = [cos(psi),sin(psi),0;
    -sin(psi),cos(psi),0;
    0,0,1];

== matlab function EOM_oceancurrents/propulsion port side/MATLAB Function7 ==
  data: T_ps_req input; rpmreq output
function rpmreq = fcn(T_ps_req)

%rpmreq = −58.37*T_ps_req^3+17.74*T_ps_req^2+756.83*T_ps_req−79.40;
rpmreq = -58.216*T_ps_req^3 + 17.943*T_ps_req^2 + 756.38*T_ps_req - 79.677

== matlab function EOM_oceancurrents/propulsion star board/MATLAB Function8 ==
  data: rpm_motor input; Thrust_sb output
function Thrust_sb  = fcn(rpm_motor)

Thrust_sb = 2E-09*rpm_motor^3 + 2E-07*rpm_motor^2 + 0.0003*rpm_motor + 0.0261;

== matlab function EOM_oceancurrents/propulsion port side/MATLAB Function9 ==
  data: rpm_motor input; Thrust_ps output
function Thrust_ps = fcn(rpm_motor)

Thrust_ps = 2E-09*rpm_motor^3 + 2E-07*rpm_motor^2 + 0.0003*rpm_motor + 0.0261;

== matlab function EOM_oceancurrents/vessel motion/C_a matrix1 ==
  data: rel_vel input; C_a output
function C_a = fcn(rel_vel)
u = rel_vel(1);
v = rel_vel(2);
r = rel_vel(3);

w = 0; % heave
p = 0; % roll
q = 0; % pitch

X_dotu = 1.2; % all of this given
X_dotv = 0;
X_dotw = 0;
X_dotp = 0;
X_dotq = 0;
X_dotr = 0;

Y_dotu = 0; 
Y_dotv = 66.1; 
Y_dotw = 0;
Y_dotp = 0;
Y_dotq = 0;
Y_dotr = 0;

a_1 = X_dotu*u + X_dotv*v +X_dotw*w + X_dotp*p + X_dotq*q +X_dotr*r;
a_2 = Y_dotu*u + Y_dotv*v +Y_dotw*w + Y_dotp*p + Y_dotq*q +Y_dotr*r;

C_a = [0,   0,   a_2;
       0,   0,  -a_1;
      -a_2, a_1,  0];

== matlab function EOM_oceancurrents/vessel motion/C_rb matrix1 ==
  data: rel_vel input; C_rb output
function C_rb = fcn(rel_vel)
u = rel_vel(1);
v = rel_vel(2);
r = rel_vel(3);

x_g = 0; % body fixed reference system located at COG
y_g = 0;
m = 18; % Mass

C_rb = [0,0, -m*(x_g*r+v);
        0,0, -m*(y_g*r-u);
        m*(x_g*r + v), m*(y_g*r- u),0];

== matlab function EOM_oceancurrents/vessel motion/D matrix1 ==
  data: rel_vel input; D output
function D = fcn(rel_vel)
u = rel_vel(1);
v = rel_vel(2);
r = rel_vel(3);

d_11 = 0.0069*u^3 - 0.1314*u^2 + 0.8842*u - 2.0431;  %X_drag
d_22 = 0.0289*v^3 - 0.5191*v^2 + 3.3058*v - 2.3601;  %Y_drag
c1 = 122.3;
c2 = 4.8;
L = 0.97;
d_33 = (1/80)*c1*r^3*L^4 + (1/12)*c2*r*L^2;

D = [d_11, 0,   0;
      0,  d_22, 0;
      0,   0,  d_33];

== matlab function EOM_oceancurrents/vessel motion/rotation matrix BODY to NED ==
  data: eta input; R output
function R = fcn(eta)
psi=eta(3);

R = [cos(psi),-sin(psi),0;
    sin(psi),cos(psi),0;
    0,0,1];

== matlab function EOM_oceancurrents/vessel motion/Rotation matrix from NED to BODY ==
  data: eta input; R output
function R = fcn(eta)
psi=eta(3);

R = [cos(psi),sin(psi),0;
    -sin(psi),cos(psi),0;
    0,0,1];

== matlab function EOM_oceancurrents/error (NED to BODY)/rotation matrix global to local ==
  data: eta input; R output
function R = fcn(eta)
psi=eta(3);

R = [cos(psi),sin(psi),0;
    -sin(psi),cos(psi),0;
    0,0,1];

== matlab function EOM_oceancurrents/vessel motion/MATLAB Function4 ==
  data: flow_B input; eta input; gamma output
function gamma = fcn(flow_B,eta)
psi=eta(3);
beta=flow_B(2);
gamma = psi-beta-pi;

== matlab function EOM_oceancurrents/vessel motion/MATLAB Function5 ==
  data: percentage input; V_body input; gamma input; F output; flow_current input
function F = fcn(percentage, V_body,gamma,flow_current)
B=0.32;
L=0.97;
rho=1000;
T_f=0.12; 
Afc=0.25*B*T_f*pi;
Alc=0.25*L*T_f*pi;

u=V_body(1);
v=V_body(2);
V=percentage/100*flow_current(3);

uc=V*cos(gamma);
vc=V*sin(gamma);

Vrc=sqrt((u-uc)^2+(v-vc)^2);
gamma_rc=-atan2((v-vc),(u-uc));
CXmax=0.48;
CYmax=0.65;
CNmax=0.065;
CX=-CXmax*cos(gamma_rc)*abs(cos(gamma_rc));
CY=CYmax*sin(gamma_rc)*abs(sin(gamma_rc));
CN=CNmax*sin(2*gamma_rc);
C=[CX;CY;CN];
Xc=0.5*rho*Afc*CX*Vrc^2;
Yc=0.5*rho*Alc*CY*Vrc^2;
Nc=0.5*rho*Alc*L*CN*Vrc^2;
F=[Xc;Yc;Nc];

== matlab function EOM_oceancurrents/vessel motion/velocity of the current in NED ==
  data: u input; vcned output; percentage input
function vcned = fcn(u, percentage)
a=u(1);
b=u(2);
c=percentage/100 * u(3);
vcned = [c*cos(a)*cos(b) ;c*sin(b); c*sin(a)*cos(b)];
